simulink model "model"  (Simulink 7.5)
settings: Solver=ode45  StartTime=0.0  StopTime=10.0  RelTol=1e-3
values from neighbouring files (symbols this model uses):
  B = J*R/psien^2    (= 0.205960224155)    [dane.m]
  In = 130.7    [dane.m]
  J = 6*Js    (= 5.82)    [dane.m]
  Kp = 1.5*Un/10    (= 66)    [dane.m]
  Kt = 10/1.2/wn    (= 0.0548810148593)    [dane.m]
  Kw = J/(2*Kt*kz*beta*psien)    [dane.m]
  m = sqrt(B*T)    [dane.m]
  psien = (Un-R*In)/wn    (= 2.67908610996)    [dane.m]
  R = 0.254    [dane.m]
  T = L/R    (= 0.00641732283465)    [dane.m]
  Un = 440    [dane.m]
  V = Kp*Y/R*B*beta/(sqrt(B*T)-beta)    [dane.m]
  Y = 10/2.5/In    (= 0.0306044376435)    [dane.m]
undefined symbols (not defined in the file or in its folder): lambdaN, Rt
settings Model: Creator=Konrad  LastModifiedBy=Konrad

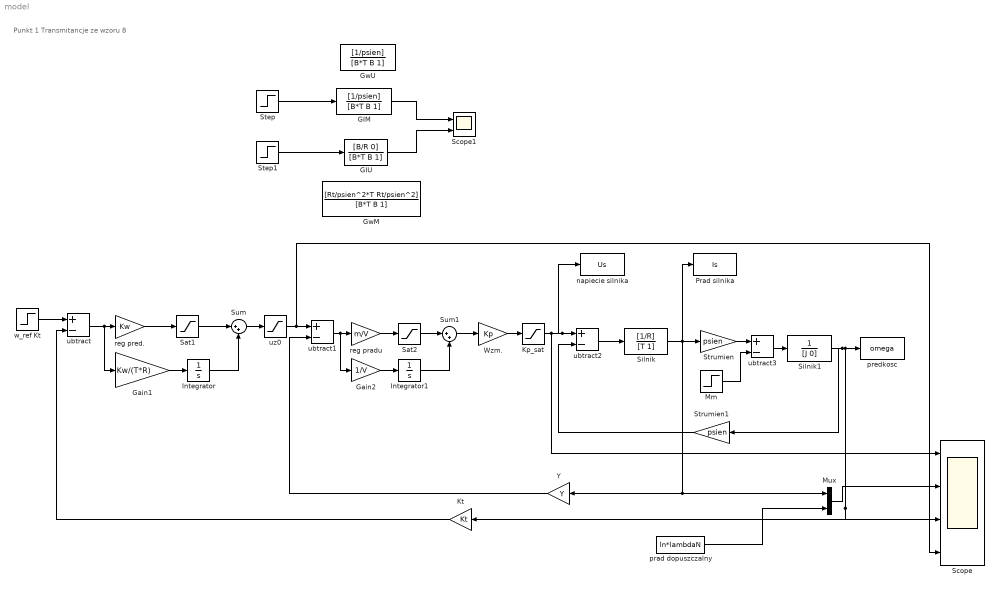
== system model ==
  note: Punkt 1
      | Transmitancje ze wzoru 8
  GIM : TransferFcn  Numerator=[1/psien]  Denominator=[B*T B 1]
  GIU : TransferFcn  Numerator=[B/R 0]  Denominator=[B*T B 1]
  Gain1 : Gain  Gain=Kw/(T*R)  ParameterDataType=fixdt(1, 16)  ParameterScaling=2^0  OutDataType=fixdt(1, 16)  OutScaling=2^0
  Gain2 : Gain  Gain=1/V  ParameterDataType=fixdt(1, 16)  ParameterScaling=2^0  OutDataType=fixdt(1, 16)  OutScaling=2^0
  GwM : TransferFcn  Numerator=[Rt/psien^2*T Rt/psien^2]  Denominator=[B*T B 1]
  GwU : TransferFcn  Numerator=[1/psien]  Denominator=[B*T B 1]
  Integrator : Integrator  LimitOutput=on  UpperSaturationLimit=1  LowerSaturationLimit=0
  Integrator1 : Integrator  LimitOutput=on  UpperSaturationLimit=1  LowerSaturationLimit=0
  Kp_sat : Saturate  OutDataType=fixdt(1, 16)  OutScaling=2^0
  Kt : Gain  Gain=Kt  ParameterDataType=fixdt(1, 16)  ParameterScaling=2^0  OutDataType=fixdt(1, 16)  OutScaling=2^0
  Mm : Step  SampleTime=0
  Mux : Mux  Inputs=2
  Prad silnika : ToWorkspace  VariableName=Is  SampleTime=-1  SaveFormat=Structure
  Sat1 : Saturate  UpperLimit=10  LowerLimit=-10  OutDataType=fixdt(1, 16)  OutScaling=2^0
  Sat2 : Saturate  UpperLimit=10  LowerLimit=-10  OutDataType=fixdt(1, 16)  OutScaling=2^0
  Scope : Scope  NumInputPorts=4
      settings: YMin=-5~-5~-5~-5  YMax=5~5~5~5
  Scope1 : Scope  NumInputPorts=2
      settings: YMin=-5~-5  YMax=5~5
  Silnik : TransferFcn  Numerator=[1/R]  Denominator=[T 1]
  Silnik1 : TransferFcn  Denominator=[J 0]
  Step : Step  After=lambdaN*In  SampleTime=0
  Step1 : Step  After=Un  SampleTime=0
  Strumien : Gain  Gain=psien  ParameterDataType=fixdt(1, 16)  ParameterScaling=2^0  OutDataType=fixdt(1, 16)  OutScaling=2^0
  Strumien1 : Gain  Gain=psien  ParameterDataType=fixdt(1, 16)  ParameterScaling=2^0  OutDataType=fixdt(1, 16)  OutScaling=2^0
  Sum : Sum  Inputs=|++  OutDataType=fixdt(1, 16)  OutScaling=2^0
  Sum1 : Sum  Inputs=|++  OutDataType=fixdt(1, 16)  OutScaling=2^0
  Wzm. : Gain  Gain=Kp  ParameterDataType=fixdt(1, 16)  ParameterScaling=2^0  OutDataType=fixdt(1, 16)  OutScaling=2^0
  Y : Gain  Gain=Y  ParameterDataType=fixdt(1, 16)  ParameterScaling=2^0  OutDataType=fixdt(1, 16)  OutScaling=2^0
  napiecie silnika : ToWorkspace  VariableName=Us  SampleTime=-1  SaveFormat=Structure
  prad dopuszczalny : FromWorkspace  VariableName=ln*lambdaN  SampleTime=0
  predkosc : ToWorkspace  VariableName=omega  SampleTime=-1  SaveFormat=Structure
  reg pradu : Gain  Gain=m/V  ParameterDataType=fixdt(1, 16)  ParameterScaling=2^0  OutDataType=fixdt(1, 16)  OutScaling=2^0
  reg pred. : Gain  Gain=Kw  ParameterDataType=fixdt(1, 16)  ParameterScaling=2^0  OutDataType=fixdt(1, 16)  OutScaling=2^0
  ubtract{,1..3} (4 alike) : Sum  Inputs=+-  OutDataType=fixdt(1, 16)  OutScaling=2^-10
  uz0 : Saturate  UpperLimit=5  LowerLimit=-5  OutDataType=fixdt(1, 16)  OutScaling=2^0
  w_ref Kt : Step  After=Un  SampleTime=0
  wires:
  w_ref Kt/1 -> ubtract/1
  ubtract/1 -> reg pred./1, Gain1/1
  reg pred./1 -> Sat1/1
  Sat1/1 -> Sum/1
  Gain1/1 -> Integrator/1
  Integrator/1 -> Sum/2
  Sum/1 -> uz0/1
  uz0/1 -> ubtract1/1, Scope/4
  ubtract1/1 -> reg pradu/1, Gain2/1
  reg pradu/1 -> Sat2/1
  Sat2/1 -> Sum1/1
  Gain2/1 -> Integrator1/1
  Integrator1/1 -> Sum1/2
  Sum1/1 -> Wzm./1
  Wzm./1 -> Kp_sat/1
  Kp_sat/1 -> ubtract2/1, napiecie silnika/1, Scope/1
  ubtract2/1 -> Silnik/1
  Silnik/1 -> Strumien/1, Prad silnika/1, Mux/1, Y/1
  Strumien/1 -> ubtract3/1
  Mm/1 -> ubtract3/2
  ubtract3/1 -> Silnik1/1
  Silnik1/1 -> Strumien1/1, predkosc/1, Scope/3, Kt/1
  Mux/1 -> Scope/2
  prad dopuszczalny/1 -> Mux/2
  Strumien1/1 -> ubtract2/2
  Y/1 -> ubtract1/2
  Kt/1 -> ubtract/2
  GIM/1 -> Scope1/1
  GIU/1 -> Scope1/2
  Step1/1 -> GIU/1
  Step/1 -> GIM/1
